simulink model "FourTanks_noControl"  (R2023b)
settings: Solver=ode4  StartTime=0.0  StopTime=1/10  FixedStep=1/10  RelTol=1e-3  EnableMultiTasking=on
InitFcn:
  | init_fourtanks
values from neighbouring files (symbols this model uses):
  gamma1 = 0.7    [init_fourtanks.m]
  gamma2 = 0.7    [init_fourtanks.m]
  gamma3 = 1.0    (= 1)    [init_fourtanks.m]
  gamma4 = 1.0    (= 1)    [init_fourtanks.m]
  gammaA = 0.6    [init_fourtanks.m]
  gammaB = 0.6    [init_fourtanks.m]
undefined symbols (not defined in the file or in its folder): u0
settings Model: Creator=Windows  LastModifiedBy=HP
settings SolverCC: AlgebraicLoopSolver=TrustRegion
settings DataIOCC: ReturnWorkspaceOutputs=off
settings OptimizationCC: DefaultParameterBehavior=Inlined  BufferReuse=off
settings DebuggingCC: UnconnectedInputMsg=warning  UnconnectedOutputMsg=warning  UnconnectedLineMsg=warning  InitInArrayFormatMsg=none  ArithmeticOperatorsInVariantConditions=warning
settings ModelReferenceCC: EnableRefExpFcnMdlSchedulingChecks=on
settings SFSimCC: CustomCodeUndefinedFunction=UseInterfaceOnly
settings RTWCC: DLArmComputeVersion=19.05

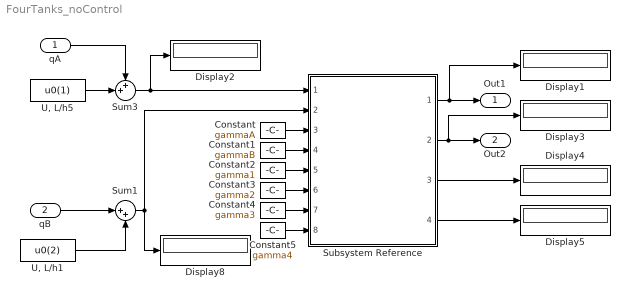
== system FourTanks_noControl ==
  qA : Inport
  qB : Inport  Port=2
  Constant : Constant  Value=gammaA
  Constant1 : Constant  Value=gammaB
  Constant2 : Constant  Value=gamma1
  Constant3 : Constant  Value=gamma2
  Constant4 : Constant  Value=gamma3
  Constant5 : Constant  Value=gamma4
  Display{1..5,8} (6 alike) : Display
  Subsystem Reference : Subsystem  ReferencedSubsystem=FourTanks_Sub
  Sum1 : Sum  Inputs=|++
  Sum3 : Sum  Inputs=++|
  "U, L/h1" : Constant  Value=u0(2)
  "U, L/h5" : Constant  Value=u0(1)
  Out1 : Outport  VectorParamsAs1DForOutWhenUnconnected=off
  Out2 : Outport  Port=2  VectorParamsAs1DForOutWhenUnconnected=off
  wires:
  Subsystem Reference/2 -> Display3/1, Out2/1
  Subsystem Reference/1 -> Display1/1, Out1/1
  Subsystem Reference/3 -> Display4/1
  Subsystem Reference/4 -> Display5/1
  Sum3/1 -> Subsystem Reference/1, Display2/1
  Sum1/1 -> Subsystem Reference/2, Display8/1
  Constant/1 -> Subsystem Reference/3
  Constant1/1 -> Subsystem Reference/4
  Constant2/1 -> Subsystem Reference/5
  Constant3/1 -> Subsystem Reference/6
  Constant4/1 -> Subsystem Reference/7
  Constant5/1 -> Subsystem Reference/8
  "U, L/h1"/1 -> Sum1/2
  qB/1 -> Sum1/1
  qA/1 -> Sum3/1
  "U, L/h5"/1 -> Sum3/2
